simulink model "pvwatts_cosimulation"  (Simulink 8.1)
settings: Solver=ode3  StartTime=0  StopTime=86400  FixedStep=1  RelTol=1e-3
undefined symbols (not defined in the file or in its folder): D1, Delta, Ts
libraries: powerlib x6, CampusEnergyModeling x6
settings Model: Creator=sfrank1  LastModifiedBy=sfrank1
settings DataIOCC: SignalLoggingSaveFormat=Dataset
settings OptimizationCC: ExpressionDepthLimit=128
settings DebuggingCC: FcnCallInpInsideContextMsg=EnableAllAsError
settings GRTTargetCC: CombineOutputUpdateFcns=on  GRTInterface=off

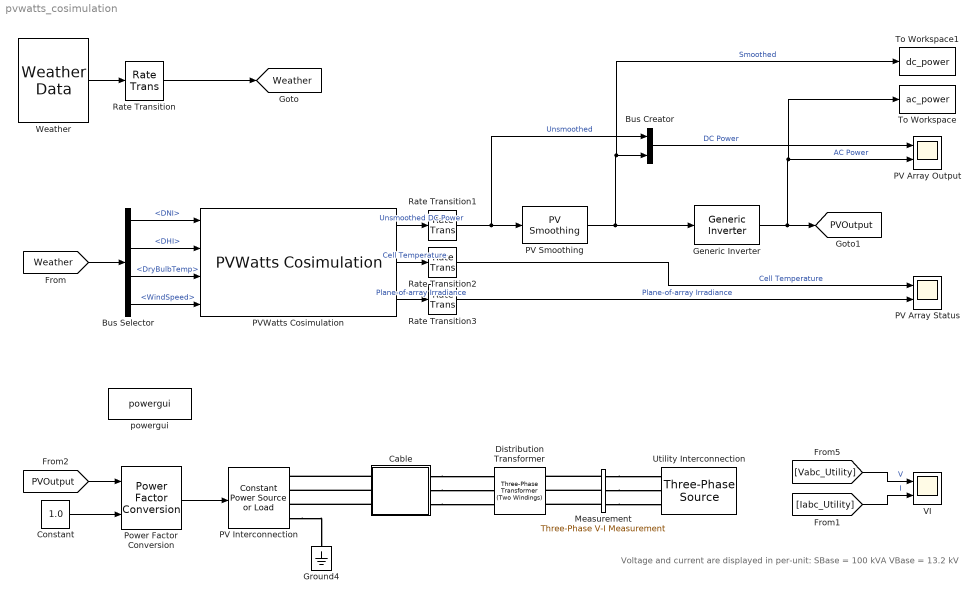
== system pvwatts_cosimulation ==
  note: Voltage and current are displayed in per-unit:
      | SBase = 100 kVA
      | VBase = 13.2 kV
  Bus Creator : BusCreator  Inputs=2
  Bus Selector : BusSelector  OutputSignals=DNI,DHI,DryBulbTemp,WindSpeed
  Cable : Subsystem  mask(Short Cable){R1=0.010, X1=0.043, R0=0.030, X0=0.129, L=500}
      mask prompts: R1 "Positive Sequence R (ohms/1000ft)"; X1 "Positive Sequence XL (ohms/1000ft)"; R0 "Zero Sequence R (ohms/1000ft)"; X0 "Zero Sequence XL (ohms/1000ft)"; L "Line Length (ft)"
      mask help:
      | This block implements a short cable using three phase mutual inductance.
      | Self impedances and mutual impedances are set by entering positive and zero sequences parameters.
      mask Display: plot(0,0,100,100,[20,20,80,80,90,80,80,20,20,10],[50,40,40,50,50,50,61,61,50,50])
  Constant : Constant  Value=1.0
  Distribution Transformer : powerlib/Elements/Three-Phase Transformer (Two Windings)  Winding1Connection=Delta (D1)  UNITS=pu  NominalPower=[100e3 , 60]  Winding1=[13.2e3 , 0.02/2 , 0.05/(120*pi)/2]  Winding2Connection=Yg  Winding2=[480 , 0.02/2 , 0.05/(120*pi)/2]  SetSaturation=off  Rm=500  Lm=200  Saturation=[ 0,0 ; 0.0024,1.2 ; 1.0,1.52 ]  Hysteresis=off  DataFile='hysteresis'  SetInitialFlux=off  InitialFluxes=[ 0.8 , -0.8 , 0.7 ]  Measurements=None  MoreParameters=off  BreakLoop=off  DataType=off  TransfoNumber=1
  Generic Inverter : CampusEnergyModeling/PV/Generic Inverter  model_type=Quadratic  fixed_eff=0.95  alpha=500  beta=4e-3  gamma=3e-7  lookup_pair=Input Power + Output Power  lookup_in=[0, 10, 25, 50, 75, 100]  lookup_out=[0, 9, 24, 49, 73, 97]  lookup_eff=[0.10, 0.80, 0.87, 0.93, 0.90, 0.88]
  Ground4 : powerlib/Elements/Ground  LConnTagsString=a
  Measurement : powerlib/Measurements/Three-Phase V-I Measurement  VoltageMeasurement=phase-to-ground  SetLabelV=on  LabelV=Vabc_Utility  Vpu=on  VpuLL=off  CurrentMeasurement=yes  SetLabelI=on  LabelI=Iabc_Utility  Ipu=on  Pbase=100e3  Vbase=13.2e3  OutputType=Magnitude  PhasorSimulation=on  PSBequivalent=0
  PV Interconnection : CampusEnergyModeling/Electrical/Constant Power Source or Load  Conven=source  PNom=100e3  QNom=0  VNom=480  fNom=60  VLow=0.7
  PV Array Output : Scope  NumInputPorts=2
      settings: ShowLegends=on  TimeRange=90000  YMin=0~-20000  YMax=140000~120000
  PV Array Status : Scope  NumInputPorts=2
      settings: ShowLegends=on  TimeRange=90000  YMin=0~0  YMax=70~1600
  PV Smoothing : CampusEnergyModeling/PV/PV Smoothing  sel=Array Size and Power Density  tc=15  area=33000  size=100e4  density=120  coverage=0.15
  PVWatts Cosimulation : CampusEnergyModeling/PV/PVWatts Cosimulation  lat=39.74  lon=-105.18  start_time=2012-06-01 00:00:00  tz=-6  time_step=10  system_size=100e3  derate=0.95  azimuth=180  tilt=39.74  use_lat_tilt=on  track_mode=Fixed  rotlim=45  use_cell_data=off  t_ref=25  t_noct=45  gamma=-0.5  i_ref=1000  poa_cutin=0  init_tcell=13.2  init_poa=0  output_dc=on  output_celltemp=on  output_poa=on
  Power Factor Conversion : CampusEnergyModeling/Electrical/Power Factor Conversion  pfType=Lagging
  Rate Transition{,1..3} (4 alike) : RateTransition  OutPortSampleTimeOpt=Inherit  OutPortSampleTime=600
  To Workspace : ToWorkspace  VariableName=ac_power  SampleTime=-1
  To Workspace1 : ToWorkspace  VariableName=dc_power  SampleTime=-1
  Utility Interconnection : powerlib/Electrical Sources/Three-Phase Source  Voltage=13.2e3  PhaseAngle=0  Frequency=60  InternalConnection=Yg  SpecifyImpedance=on  Resistance=0.8929  Inductance=16.58e-3  ShortCircuitLevel=1e6  BaseVoltage=13.2e3  XRratio=8  BusType=swing  Pref=0  Qref=0  Qmin=-inf  Qmax=inf
  VI : Scope  NumInputPorts=2
      settings: ShowLegends=on  TimeRange=90000  YMin=0.999~0  YMax=1.007~1.4  SaveName=ScopeData2
  Weather : CampusEnergyModeling/Weather/Weather Data  fname=Weather-short.mat  initbus=on
  powergui : powerlib/powergui  Priority=2  SimulationMode=Phasor  SolverType=Tustin  SampleTime=Ts  frequency=60  SPID=off  DisableSnubberDevices=off  DisableRonSwitches=off  DisableVfSwitches=off  SwTol=0  Interpol=off  DisplayEquations=off  frequencyindice=60  Pbase=100e6  ErrMax=1e-4  Iterations=50  UnitsV=kV  UnitsW=kW  FunctionMessages=off  echomessages=off  HookPort=off  EnableUseOfTLC=off  x0status=blocks  RestoreLinks=warning  ResistiveCurrentMeasurement=off  Frange=[0:2:500]  Ylog=off  Xlog=on  ShowGrid=off  save=off  variable=ZData  structure=Sig1  ZoomFFT=on  StartTime=0.26  cycles=2  DisplayStyle=1  fundamental=60  FreqAxis=off  MaxFrequency=5000  frequencyindicesteady=1  RmsSteady=1  display=off  Ts=0  methode=off
  tag scope: PVOutput=global, Weather=global
  wires:
  PVWatts Cosimulation/1 -> Rate Transition1/1  "Unsmoothed DC Power"
  Weather/1 -> Rate Transition/1
  Bus Selector/1 -> PVWatts Cosimulation/1  "<DNI>"
  Bus Selector/2 -> PVWatts Cosimulation/2  "<DHI>"
  Bus Selector/3 -> PVWatts Cosimulation/3  "<DryBulbTemp>"
  Bus Selector/4 -> PVWatts Cosimulation/4  "<WindSpeed>"
  Rate Transition/1 -> [Weather]
  Generic Inverter/1 -> [PVOutput], To Workspace/1, PV Array Output/2  "AC Power"
  [Weather] -> Bus Selector/1
  PV Smoothing/1 -> Generic Inverter/1, To Workspace1/1, Bus Creator/2  "Smoothed"
  Rate Transition1/1 -> PV Smoothing/1, Bus Creator/1  "Unsmoothed"
  PVWatts Cosimulation/2 -> Rate Transition2/1  "Cell Temperature"
  PVWatts Cosimulation/3 -> Rate Transition3/1  "Plane-of-array Irradiance"
  Constant/1 -> Power Factor Conversion/2
  Power Factor Conversion/1 -> PV Interconnection/1
  [Vabc_Utility] -> VI/1  "V"
  [Iabc_Utility] -> VI/2  "I"
  Bus Creator/1 -> PV Array Output/1  "DC Power"
  Rate Transition2/1 -> PV Array Status/1  "Cell Temperature"
  Rate Transition3/1 -> PV Array Status/2  "Plane-of-array Irradiance"
  [PVOutput] -> Power Factor Conversion/1
  connections:
  PV Interconnection/RConn4 -- Ground4/LConn1
  Cable/RConn1 -- PV Interconnection/RConn1
  Cable/RConn2 -- PV Interconnection/RConn2
  Cable/RConn3 -- PV Interconnection/RConn3
  Cable/LConn1 -- Distribution Transformer/RConn1
  Cable/LConn2 -- Distribution Transformer/RConn2
  Cable/LConn3 -- Distribution Transformer/RConn3
  Measurement/RConn1 -- Distribution Transformer/LConn1
  Measurement/RConn2 -- Distribution Transformer/LConn2
  Measurement/RConn3 -- Distribution Transformer/LConn3
  Measurement/LConn1 -- Utility Interconnection/RConn1
  Measurement/LConn2 -- Utility Interconnection/RConn2
  Measurement/LConn3 -- Utility Interconnection/RConn3

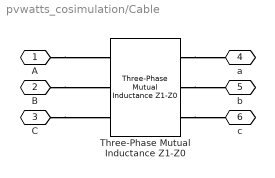
== system pvwatts_cosimulation/Cable ==
  Three-Phase Mutual Inductance Z1-Z0 : powerlib/Elements/Three-Phase Mutual Inductance Z1-Z0  LConnTagsString=a|b|c  RConnTagsString=A|B|C  PositiveSequence=[R1 X1/376.9911]*L/1000  ZeroSequence=[R0 X0/376.9911]*L/1000
  A : PMIOPort  Port=1  Side=Left
  B : PMIOPort  Port=2  Side=Left
  "C " : PMIOPort  Port=3  Side=Left
  a : PMIOPort  Port=4  Side=Right
  b : PMIOPort  Port=5  Side=Right
  c : PMIOPort  Port=6  Side=Right
  connections:
  A/RConn1 -- Three-Phase Mutual Inductance Z1-Z0/LConn1
  B/RConn1 -- Three-Phase Mutual Inductance Z1-Z0/LConn2
  "C "/RConn1 -- Three-Phase Mutual Inductance Z1-Z0/LConn3
  Three-Phase Mutual Inductance Z1-Z0/RConn1 -- a/RConn1
  Three-Phase Mutual Inductance Z1-Z0/RConn2 -- b/RConn1
  Three-Phase Mutual Inductance Z1-Z0/RConn3 -- c/RConn1
